simulink model "Model_nanoCT_2_hysteresis_OST_Nam"  (R2017a)
settings: Solver=ode23t  StartTime=0.0  StopTime=0.21  MaxStep=1e-4  RelTol=1e-3  EnableMultiTasking=on
values from neighbouring files (symbols this model uses):
  f = f(ind_beg:ind_end)    [Freq_estimation.m]    (also in Frequency_estimation_1.m = 52; matlab_Kad.mat = 50)
  I = H*2*pi*((d1+d2)/4)/w1    [Calc_hysteresis.m]    (also in matlab_Kad.mat = 150)
  Lsr = 0.20106192983    [matlab_Kad.mat]
  S = h*(d1-d2)/2    (= 0.0001875)    [Calc_hysteresis.m]    (also in Parameters.m = 0.000425; matlab_Kad.mat = 0.000425)
  w1 = 1    [Calc_hysteresis.m]    (also in Parameters.m; matlab_Kad.mat)
  w2 = 10    [Calc_hysteresis.m]    (also in Parameters.m = 120; matlab_Kad.mat = 120)
libraries: fl_lib x9, nesl_utility x5, pe_lib x1, simulink x1
settings Model: Creator=Андрей  LastModifiedBy=Aleksey
settings SolverCC: ZeroCrossAlgorithm=Adaptive
settings OptimizationCC: LifeSpan=inf
settings DebuggingCC: SFUnexpectedBacktrackingDiag=warning  SFNoUnconditionalDefaultTransitionDiag=warning  SFExecutionAtInitializationDiag=none
settings GRTTargetCC: TargetLangStandard=C89/C90 (ANSI)  GeneratePreprocessorConditionals=Disable all
settings ConfigComp: CovMetricSettings=dw  CovHtmlReporting=on  CovSaveCumulativeToWorkspaceVar=on  CovSaveSingleToWorkspaceVar=on  CovExternalEMLEnable=off

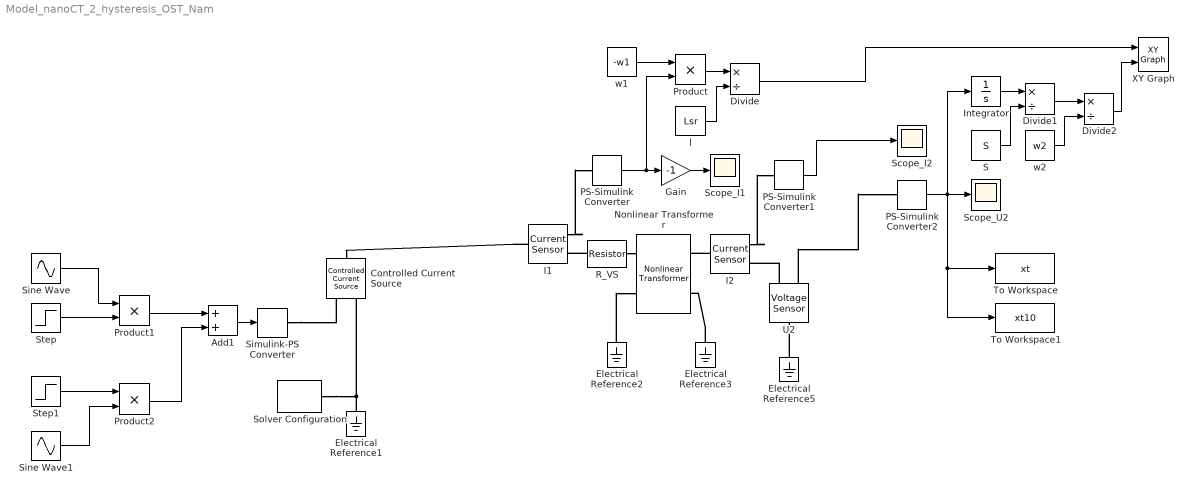
== system Model_nanoCT_2_hysteresis_OST_Nam ==
  Add1 : Sum
  Controlled Current Source : fl_lib/Electrical/Electrical Sources/Controlled Current Source
  Divide : Product  Inputs=*/
  Divide1 : Product  Inputs=*/
  Divide2 : Product  Inputs=*/
  Electrical Reference{1..3,5} (4 alike) : fl_lib/Electrical/Electrical Elements/Electrical Reference
  Gain : Gain  Gain=-1
  I1 : fl_lib/Electrical/Electrical Sensors/Current Sensor
  I2 : fl_lib/Electrical/Electrical Sensors/Current Sensor
  Integrator : Integrator
  Nonlinear Transformer : pe_lib/Passive Devices/Fundamental Components/Nonlinear Transformer  Nw=w1  Nw2=w2  winding_param_option=2  Req=0.01 Ohm  Leq=1e-4 H  R_1=0.01 Ohm  L_1=1e-4 H  R_2=R Ohm  L_2=L H  R_m=100 Ohm  parameterization_option=5  H_data=[0 200 400 600 800 1000 ] A/m  B_data=[ 0 0.81 1.25 1.42 1.48 1.49 ] T  length_effective=Lsr m  area_effective=S m^2  L=0.04 H  L_sat=0.01 H  current_data=[ 0 0.4 0.8 1.2 1.6 2 ] A  magnetic_flux_data=[ 0 0.161 0.25 0.284 0.295 0.299 ].*1e-3 Wb  magnetic_flux_sat=1.6e-4 Wb  dBdH0=0.7 m*T/A  B1=0.89 T  H1=2.82 A/m  c=0.1  K=1.2 A/m  alpha=1e-7  Leq_i0=0 A  L1_i0=0 A  L2_i0=0 A  x0_option=1  i_L0=0 A  phi0=0 Wb  B0=0 T  H0=0 A/m  Leq_g=0 1/Ohm  L1_g=1e-9 1/Ohm  L2_g=1e-9 1/Ohm  interpolation_option=2
      settings: SourceProductName=Simscape Power Systems  SourceProductBaseCode=PS
  PS-Simulink Converter : nesl_utility/PS-Simulink Converter  PhysicalDomain=network_engine_domain  SubClassName=ps_output  LeftPortType=input  RightPortType=output  PseudoPeriodic=off  Frequencies=[]  Unit=1  AffineConversion=off
  PS-Simulink Converter1 : nesl_utility/PS-Simulink Converter  PhysicalDomain=network_engine_domain  SubClassName=ps_output  LeftPortType=input  RightPortType=output  PseudoPeriodic=off  Frequencies=[]  Unit=1  AffineConversion=off
  PS-Simulink Converter2 : nesl_utility/PS-Simulink Converter  PhysicalDomain=network_engine_domain  SubClassName=ps_output  LeftPortType=input  RightPortType=output  PseudoPeriodic=off  Frequencies=[]  Unit=1  AffineConversion=off
  Product : Product
  Product1 : Product
  Product2 : Product
  R_VS : fl_lib/Electrical/Electrical Elements/Resistor  R=1 Ohm  i_specify=off  i_priority=None  i=0 A  i_nominal_specify=off  i_nominal_unit=A  i_nominal_value=1  v_specify=off  v_priority=None  v=0 V  v_nominal_specify=off  v_nominal_unit=V  v_nominal_value=1
  S : Constant  Value=S
  Scope_I1 : Scope
  Scope_I2 : Scope
  Scope_U2 : Scope
  Simulink-PS Converter : nesl_utility/Simulink-PS Converter  PhysicalDomain=network_engine_domain  SubClassName=ps_input  LeftPortType=input  RightPortType=output  PseudoPeriodic=off  Frequencies=[]  NoiseDistribution=none  NoiseParameters=[]  Unit=1  AffineConversion=off  FilteringAndDerivatives=provide  SimscapeFilterOrder=1  InputFilterTimeConstant=0.001  UdotUserProvided=0
  Sine Wave : Sin  Amplitude=I  Frequency=pi*f  Phase=pi  SampleTime=0
  Sine Wave1 : Sin  Amplitude=I/1000  Frequency=pi*f  Phase=pi  SampleTime=0
  Solver Configuration : nesl_utility/Solver Configuration  PhysicalDomain=network_engine_domain  SubClassName=solver  LeftPortType=input  RightPortType=generic  Accelerate=off  Tones=[]  Harmonics=[]  SimulateNoise=off  Profile=off  UseLocalSampling=off  EnableSwitchedLinearOptims=on  FrequencyDomain=off  UseCCode=off  RelTol=0.001  AbsTol=1e-06  MinStep=1e-09  ToWorkspace=off  RevertToSquareIcSolve=off  NumHomotopyIterations=100  PhasorMode=off  PhasorModeNumHarmonics=1  OverrideAbsTol=off  DoDC=on  ResidualTolerance=1e-09  UseLocalSolver=off  LocalSolverChoice=NE_BACKWARD_EULER_ADVANCER  LocalSolverSampleTime=0.000001  DoFixedCost=off  MaxNonlinIter=3  MaxModeIter=2  LinearAlgebra=Sparse  DelaysMemoryBudget=1024  AutomaticFiltering=off  FilteringTimeConstant=0.001
  Step : Step  Time=50e-3  Before=1  After=0  SampleTime=0
  Step1 : Step  Time=60e-3  SampleTime=0
  To Workspace : ToWorkspace  VariableName=xt  SampleTime=1/f/N
      settings: MaxDataPoints=N
  To Workspace1 : ToWorkspace  VariableName=xt10  SampleTime=1/f/N
      settings: MaxDataPoints=N*10
  U2 : fl_lib/Electrical/Electrical Sensors/Voltage Sensor
  XY Graph : simulink/Sinks/XY Graph  xmin=-5  xmax=5  ymin=-1.2  ymax=1.2  st=-1
  l : Constant  Value=Lsr
  w1 : Constant  Value=-w1
  w2 : Constant  Value=w2
  wires:
  PS-Simulink Converter/1 -> Gain/1, Product/2
  PS-Simulink Converter2/1 -> To Workspace/1, To Workspace1/1, Scope_U2/1, Integrator/1
  PS-Simulink Converter1/1 -> Scope_I2/1
  w1/1 -> Product/1
  Product/1 -> Divide/1
  l/1 -> Divide/2
  Integrator/1 -> Divide1/1
  S/1 -> Divide1/2
  Divide1/1 -> Divide2/1
  w2/1 -> Divide2/2
  Divide2/1 -> XY Graph/2
  Divide/1 -> XY Graph/1
  Product1/1 -> Add1/1
  Sine Wave/1 -> Product1/1
  Step/1 -> Product1/2
  Add1/1 -> Simulink-PS Converter/1
  Sine Wave1/1 -> Product2/2
  Step1/1 -> Product2/1
  Product2/1 -> Add1/2
  Gain/1 -> Scope_I1/1
  connections:
  I2/LConn1 -- Nonlinear Transformer/RConn1
  U2/RConn2 -- I2/RConn2
  I1/RConn1 -- PS-Simulink Converter/LConn1
  I2/RConn1 -- PS-Simulink Converter1/LConn1
  U2/RConn1 -- PS-Simulink Converter2/LConn1
  R_VS/RConn1 -- I1/RConn2
  R_VS/LConn1 -- Nonlinear Transformer/LConn1
  Electrical Reference1/LConn1 -- Controlled Current Source/RConn2 -- Solver Configuration/RConn1
  Electrical Reference2/LConn1 -- Nonlinear Transformer/LConn2
  Electrical Reference3/LConn1 -- Nonlinear Transformer/RConn2
  Electrical Reference5/LConn1 -- U2/LConn1
  I1/LConn1 -- Controlled Current Source/LConn1
  Simulink-PS Converter/RConn1 -- Controlled Current Source/RConn1
